simulink model "Plant"  (R2020b)
settings: Solver=VariableStepAuto  StartTime=0.0  StopTime=10.0  RelTol=1e-3
PreLoadFcn:
  | b = 50;
  | m = 1000;
  | u = 500;
settings Model: Creator=sai  LastModifiedBy=sai

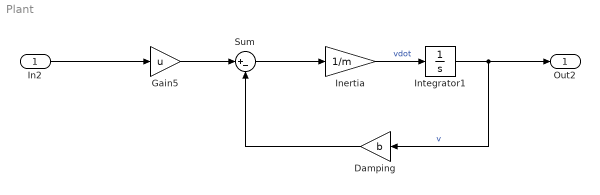
== system Plant ==
  In2 : Inport  OutDataTypeStr=double  PortDimensions=1  SampleTime=0
  Damping : Gain  Gain=b
  Gain5 : Gain  Gain=u
  Inertia : Gain  Gain=1/m
  Integrator1 : Integrator
  Sum : Sum  Inputs=|+-
  Out2 : Outport  OutDataTypeStr=double  PortDimensions=1  SampleTime=0
  wires:
  Damping/1 -> Sum/2
  Integrator1/1 -> Damping/1, Out2/1  "v"
  Gain5/1 -> Sum/1
  In2/1 -> Gain5/1
  Inertia/1 -> Integrator1/1  "vdot"
  Sum/1 -> Inertia/1
